simulink library "Feuchtesimulation_Lib"  (R2018b)
settings: Solver=VariableStepAuto  StartTime=0.0  StopTime=10.0  RelTol=1e-3
undefined symbols (not defined in the file or in its folder): A_Kat0, A_Mantel_Kat0, Ads_AusnutzungsFaktor, adsorptionsenthalpie, AIR_mw, beladungskennfeld, c_edelstahl, c_Isomatte, deltaH_verd, DiscIntNeverNeededParam, H2O_mw, Kat0_Anzahl_Zonen, Kond_AusnutzungsFaktor, Kond_KL_Faktor_, KondVerd_KLKF_mf_StSt_kgps, l_Kat0, m_Canning_Kat0, m_h2o_kat0_ads, m_h2o_kat0_kond, m_Isolierung_Kat0, m_zeolith_kat0_zone, m_zKat0, Mat_Kat0, mGas_imRohrabschnitt_kg, mZeo_UnterDerZeo0angenommenWird, p_dsat, R_sLuft, rate_k_verd, Rohr1, RTh_Brick_Iso_Kat0, RTh_Iso_Canning_Kat0, Sensor0, SensorIn, switch_TInit_Tstart_bei_true_sonst_TInitAusMessung, T_start, Tk0_1, ts, Verd_KF_Dampfdruck_StSt, Verd_KL_Faktor, waermekapazitaet_luft, waermekapazitaet_wasser_fluessig, waermekapazitaet_wasser_gasfoermig, WuezRohr_Dynamikfaktor
libraries: simulink x5, $bdroot x3
(part 2 of 2)

== system Feuchtesimulation_Lib/Brick/Adsorption Kondensation/Eingangskorrektur Adsorption ==
  note: Da das Adsorptionsmodell nachgeschalten ist kann es sein, dass das Model Wasser
      | "austragen" möchte obwohl kein Kondenzwasser verfügbar ist.
      |
      | Wenn m_Kond<=0 und deltaS<0 (sF kleiner als maximale Feuchte), dann ist der
      | Ausgang 0
  Delta S Kondensation : Inport
  Masse Kondensation : Inport  Port=2
  Constant2 : Constant  Value=0
  MATLAB Function : MATLAB Function  TreatAsAtomicUnit=on
  Switch : Switch  Criteria=u2 > Threshold
  Korrektur Adsorption Eingang : Outport
  wires:
  Delta S Kondensation/1 -> Switch/3, MATLAB Function/1(u1)
  Constant2/1 -> Switch/1
  MATLAB Function/1(y) -> Switch/2
  Masse Kondensation/1 -> MATLAB Function/2(u2)
  Switch/1 -> Korrektur Adsorption Eingang/1

== system Feuchtesimulation_Lib/Brick/Adsorption Kondensation/Kondensation ==
  note: Berechnet die Maximale Feuchte über die Formel:
      | s_max = H2O_mw/AIR_mw*p_dsat/(p-(1-H2O_mw/AIR_mw)*p_dsat)
      |
      | Der sättigungsdampfdruck wird über das Kennfeld bestimmt
  Bauteiltemperatur [°C] : Inport
  Druck [mbar] : Inport  Port=2
  spezifische Feuchte [kg/kg] : Inport  Port=3
  1-D Lookup Table : Lookup_n-D  NumberOfTableDimensions=1  BreakpointsForDimension1=p_dsat.T  Table=p_dsat.p  ExtrapMethod=Clip  InternalRulePriority=Speed  RndMeth=Simplest  InputSameDT=on
  Gain : Gain  Gain=Kond_AusnutzungsFaktor
  Limit Sättigungsdampfdruck : Subsystem
  Maximale spez Luftf. : MATLAB Function  TreatAsAtomicUnit=on
  Sat 0-1 : Saturate  UpperLimit=1  LowerLimit=0
  Sum : Sum  Inputs=|+-
  Ueberschuss spez. Feuchte [kg/kg] : Outport
  wires:
  1-D Lookup Table/1 -> Limit Sättigungsdampfdruck/2(Sättigungsdampfdruck [mbar])
  Bauteiltemperatur [°C]/1 -> 1-D Lookup Table/1
  Maximale spez Luftf./1(s_max) -> Sat 0-1/1
  Sum/1 -> Gain/1
  spezifische Feuchte [kg/kg]/1 -> Sum/1
  Sat 0-1/1 -> Sum/2
  Limit Sättigungsdampfdruck/1(Sättigungsdampfdruck Limitiert [mbar]) -> Maximale spez Luftf./2(p_dsat_mbar)
  Druck [mbar]/1 -> Limit Sättigungsdampfdruck/1(Druck [mbar]), Maximale spez Luftf./1(p_mbar)
  Gain/1 -> Ueberschuss spez. Feuchte [kg/kg]/1

== system Feuchtesimulation_Lib/Brick/Adsorption Kondensation/Theta Max  ==
  note: Ermittelt die aktuell maximal mögliche Wasserbeladung des Zeolithmasse
      | in Abhängigkeit der Temperatur und des Wasserdampfpartialdrucks
  Bauteiltemperatur [°C] : Inport
  Druck in [mbar] : Inport  Port=2
  spezifische Feuchte [kg/kg] : Inport  Port=3
  % to 1 : Gain  Gain=0.01
  2-D Lookup Table : Lookup_n-D  BreakpointsForDimension1=beladungskennfeld.Temp_C  BreakpointsForDimension2=beladungskennfeld.pSat_Pa  Table=beladungskennfeld.Beladung_prz  ExtrapMethod=Clip  InternalRulePriority=Speed  RndMeth=Simplest  InputSameDT=on
  S to E : Subsystem  AncestorBlock=Kats/S to E
  mbar to pa : Gain  Gain=100
  Theta_max [kg/kg] : Outport
  wires:
  mbar to pa/1 -> 2-D Lookup Table/2
  % to 1/1 -> Theta_max [kg/kg]/1
  2-D Lookup Table/1 -> % to 1/1
  spezifische Feuchte [kg/kg]/1 -> S to E/2(s)
  Druck in [mbar]/1 -> S to E/1(p_mbar)
  Bauteiltemperatur [°C]/1 -> 2-D Lookup Table/1
  S to E/1(e_mbar) -> mbar to pa/1

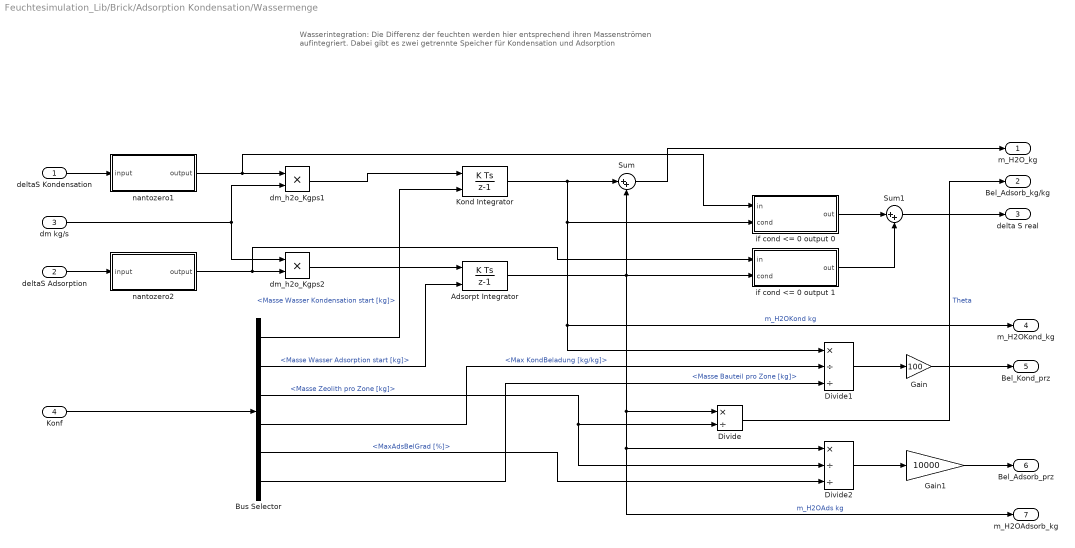
== system Feuchtesimulation_Lib/Brick/Adsorption Kondensation/Wassermenge  ==
  note: Wasserintegration:
      | Die Differenz der feuchten werden hier entsprechend ihren Massenströmen aufintegriert.
      | Dabei gibt es zwei getrennte Speicher für Kondensation und Adsorption
  deltaS Kondensation : Inport
  deltaS Adsorption : Inport  Port=2
  dm kg/s : Inport  Port=3
  Konf : Inport  Port=4
  Adsorpt Integrator : DiscreteIntegrator  InitialConditionSource=external  SampleTime=ts  LimitOutput=on  LowerSaturationLimit=0  ICPrevOutput=DiscIntNeverNeededParam  ICPrevScaledInput=DiscIntNeverNeededParam
  Bus Selector : BusSelector  OutputSignals=Masse Wasser Kondensation start [kg],Masse Wasser Adsorption start [kg],Masse Zeolith pro Zone [kg],Material Bauteil.Max KondBeladung [kg/kg],Material Bauteil.MaxAdsBelGrad [%],Masse Bauteil pro Zone [kg]
  Divide : Product  Inputs=*/
  Divide1 : Product  Inputs=*//
  Divide2 : Product  Inputs=*//
  Gain : Gain  Gain=100
  Gain1 : Gain  Gain=10000
  Kond Integrator : DiscreteIntegrator  InitialConditionSource=external  SampleTime=ts  LimitOutput=on  LowerSaturationLimit=0  ICPrevOutput=DiscIntNeverNeededParam  ICPrevScaledInput=DiscIntNeverNeededParam
  Sum : Sum  Inputs=|++
  Sum1 : Sum  Inputs=|++
  dm_h2o_Kgps1 : Product
  dm_h2o_Kgps2 : Product
  if cond <= 0 output 0 : Subsystem
  if cond <= 0 output 1 : Subsystem
  nantozero1 : Subsystem
  nantozero2 : Subsystem
  m_H2O_kg : Outport
  Bel_Adsorb_kg/kg : Outport  Port=2
  delta S real : Outport  Port=3
  m_H2OKond_kg : Outport  Port=4
  Bel_Kond_prz : Outport  Port=5
  Bel_Adsorb_prz : Outport  Port=6
  m_H2OAdsorb_kg : Outport  Port=7
  wires:
  deltaS Kondensation/1 -> nantozero1/1(input)
  deltaS Adsorption/1 -> nantozero2/1(input)
  Bus Selector/3 -> Divide2/2, Divide/2  "<Masse Zeolith pro Zone [kg]>"
  Divide/1 -> Bel_Adsorb_kg/kg/1  "Theta"
  Sum/1 -> m_H2O_kg/1
  dm_h2o_Kgps1/1 -> Kond Integrator/1
  dm_h2o_Kgps2/1 -> Adsorpt Integrator/1
  dm kg/s/1 -> dm_h2o_Kgps1/2, dm_h2o_Kgps2/1
  Kond Integrator/1 -> Divide1/1, m_H2OKond_kg/1, if cond <= 0 output 0/2(cond), Sum/1  "m_H2OKond kg"
  Sum1/1 -> delta S real/1
  Adsorpt Integrator/1 -> if cond <= 0 output 1/2(cond), m_H2OAdsorb_kg/1, Divide2/1, Divide/1, Sum/2  "m_H2OAds kg"
  nantozero2/1(output) -> if cond <= 0 output 1/1(in), dm_h2o_Kgps2/2
  Konf/1 -> Bus Selector/1
  Bus Selector/2 -> Adsorpt Integrator/2  "<Masse Wasser Adsorption start [kg]>"
  Bus Selector/1 -> Kond Integrator/2  "<Masse Wasser Kondensation start [kg]>"
  if cond <= 0 output 0/1(out) -> Sum1/1
  if cond <= 0 output 1/1(out) -> Sum1/2
  Divide1/1 -> Gain/1
  Bus Selector/4 -> Divide1/2  "<Max KondBeladung [kg/kg]>"
  nantozero1/1(output) -> if cond <= 0 output 0/1(in), dm_h2o_Kgps1/1
  Bus Selector/5 -> Divide2/3  "<MaxAdsBelGrad [%]>"
  Gain/1 -> Bel_Kond_prz/1
  Divide2/1 -> Gain1/1
  Gain1/1 -> Bel_Adsorb_prz/1
  Bus Selector/6 -> Divide1/3  "<Masse Bauteil pro Zone [kg]>"

== system Feuchtesimulation_Lib/Brick/Enthalpiestrom ausgehend /kombinierte Wärmekapazität ==
  Spezifische Feuchte : Inport
  Constant : Constant
  Constant1 : Constant  Value=waermekapazitaet_wasser_gasfoermig
  Multiply : Product
  Multiply1 : Product
  Sum : Sum  Inputs=|+-
  Sum1 : Sum  Inputs=|++
  cp1 : Constant  Value=waermekapazitaet_luft
  kombinierte Wärmekapazität : Outport
  wires:
  Multiply/1 -> Sum1/2
  Sum/1 -> Multiply/1
  Constant/1 -> Sum/1
  Spezifische Feuchte/1 -> Sum/2, Multiply1/1
  Constant1/1 -> Multiply1/2
  cp1/1 -> Multiply/2
  Multiply1/1 -> Sum1/1
  Sum1/1 -> kombinierte Wärmekapazität/1

== system Feuchtesimulation_Lib/Brick/Enthalpiestrom eingehend /kombinierte Wärmekapazität ==
  Spezifische Feuchte : Inport
  Constant : Constant
  Constant1 : Constant  Value=waermekapazitaet_wasser_gasfoermig
  Multiply : Product
  Multiply1 : Product
  Sum : Sum  Inputs=|+-
  Sum1 : Sum  Inputs=|++
  cp1 : Constant  Value=waermekapazitaet_luft
  kombinierte Wärmekapazität : Outport
  wires:
  Multiply/1 -> Sum1/2
  Sum/1 -> Multiply/1
  Constant/1 -> Sum/1
  Spezifische Feuchte/1 -> Sum/2, Multiply1/1
  Constant1/1 -> Multiply1/2
  cp1/1 -> Multiply/2
  Multiply1/1 -> Sum1/1
  Sum1/1 -> kombinierte Wärmekapazität/1

== system Feuchtesimulation_Lib/Rohrwandabschnitt/Kondensation/Taupunkt ==
  note: Berechnet die Taupunkttemperatur abhängig von abs. Druck und Feuchte
      |
      | TP-Formel basiert auf Magnusformel für Sättigungsdampfdruck
      | (Gültigkeitsbereich -45 (unterkühltes Wasser) bis +60°C, passt aber gut für
      | alle sinnvoll überprüften Werte) und benötigt neben dem absoluten Druck
      | als Feuchtemaß das Mischungsverhältnis (mWasser/mtrockeneLuft, 0 - inf),
      | welches sF/(1-sF) ist.
  spezifische Feuchte [kg/kg] : Inport
  Druck [mbar] : Inport  Port=2
  0<x<=0.999 : Saturate  UpperLimit=0.999  LowerLimit=0
  1e-6<x<1e6 : Saturate  UpperLimit=1e6  LowerLimit=1e-6
  Constant2 : Constant
  MATLAB Function : MATLAB Function  TreatAsAtomicUnit=on
  Sum : Sum  Inputs=-+
  sF/(1-sF) : Product  Inputs=*/
  Taupunkt [°C] : Outport
  wires:
  MATLAB Function/1(T_tp) -> Taupunkt [°C]/1
  Druck [mbar]/1 -> MATLAB Function/2(p)
  Constant2/1 -> Sum/2
  Sum/1 -> sF/(1-sF)/2
  sF/(1-sF)/1 -> 1e-6<x<1e6/1  "Mischungsverhaeltnis x"
  0<x<=0.999/1 -> Sum/1, sF/(1-sF)/1
  spezifische Feuchte [kg/kg]/1 -> 0<x<=0.999/1
  1e-6<x<1e6/1 -> MATLAB Function/1(x)

== system Feuchtesimulation_Lib/Rohrwandabschnitt/Q Gas an Wand/dm_2_v ==
  dm_kg/s : Inport
  p_mbar : Inport  Port=2
  Tg_C : Inport  Port=3
  D_eff_m : Inport  Port=4
  A_Rohr_m2 : Product  Inputs=***
  Constant1 : Constant  Value=3.14/4
  Constant2 : Constant  Value=R_sLuft
  Pa : Gain  Gain=100
  degC --> K : Subsystem
  m/A/rho : Product  Inputs=*//
  rho : Product  Inputs=*//
  v_m/s : Outport
  wires:
  dm_kg/s/1 -> m/A/rho/1
  rho/1 -> m/A/rho/2  "kg/m3"
  A_Rohr_m2/1 -> m/A/rho/3
  m/A/rho/1 -> v_m/s/1
  Constant2/1 -> rho/3
  degC --> K/1(K) -> rho/2
  p_mbar/1 -> Pa/1
  Pa/1 -> rho/1
  D_eff_m/1 -> A_Rohr_m2/2, A_Rohr_m2/1
  Constant1/1 -> A_Rohr_m2/3
  Tg_C/1 -> degC --> K/1(degC)

== system Feuchtesimulation_Lib/Brick/Adsorption Kondensation/Kondensation/Limit Sättigungsdampfdruck ==
  note: Hier wird der Maximale Sättigungsdampfdruck limitiert, da sonst in der
      | berechnung eine Singularität auftritt. Ist der Sättigungsdampfdruck gleich
      | dem Druck, ist der maximale Feuchtegehalt erreicht.
  Druck [mbar] : Inport
  Sättigungsdampfdruck [mbar] : Inport  Port=2
  Sum : Sum  Inputs=|+-
  Switch : Switch  Criteria=u2 > Threshold  RndMeth=Simplest  SaturateOnIntegerOverflow=on  InputSameDT=on
  Sättigungsdampfdruck Limitiert [mbar] : Outport
  wires:
  Druck [mbar]/1 -> Switch/3, Sum/1
  Sättigungsdampfdruck [mbar]/1 -> Switch/1, Sum/2
  Sum/1 -> Switch/2
  Switch/1 -> Sättigungsdampfdruck Limitiert [mbar]/1

== system Feuchtesimulation_Lib/Brick/Adsorption Kondensation/Theta Max /S to E ==
  p_mbar : Inport
  s : Inport  Port=2
  Constant : Constant  Value=H2O_mw/AIR_mw
  Divide : Product  Inputs=*/
  Multiply : Product
  Multiply1 : Product
  Sum : Sum  Inputs=++-
  e_mbar : Outport
  wires:
  Divide/1 -> e_mbar/1
  Sum/1 -> Divide/2
  Constant/1 -> Multiply1/2, Sum/2
  Multiply1/1 -> Sum/3
  Multiply/1 -> Divide/1
  p_mbar/1 -> Multiply/1
  s/1 -> Multiply/2, Sum/1, Multiply1/1

== system Feuchtesimulation_Lib/Brick/Adsorption Kondensation/Wassermenge /if cond <= 0 output 0 ==
  in : Inport
  cond : Inport  Port=2
  Constant : Constant  Value=0
  Switch : Switch  Criteria=u2 > Threshold  RndMeth=Simplest  SaturateOnIntegerOverflow=on  InputSameDT=on
  out : Outport
  wires:
  cond/1 -> Switch/2
  Switch/1 -> out/1
  in/1 -> Switch/1
  Constant/1 -> Switch/3

== system Feuchtesimulation_Lib/Brick/Adsorption Kondensation/Wassermenge /if cond <= 0 output 1 ==
  in : Inport
  cond : Inport  Port=2
  Constant : Constant  Value=0
  Switch : Switch  Criteria=u2 > Threshold  RndMeth=Simplest  SaturateOnIntegerOverflow=on  InputSameDT=on
  out : Outport
  wires:
  cond/1 -> Switch/2
  Switch/1 -> out/1
  in/1 -> Switch/1
  Constant/1 -> Switch/3

== system Feuchtesimulation_Lib/Brick/Adsorption Kondensation/Wassermenge /nantozero1 ==
  input : Inport
  IsNaN : RelationalOperator  Operator=isNaN  OutDataTypeStr=boolean  RndMeth=Simplest
  Switch : Switch  Criteria=u2 > Threshold
  Zero : Constant  Value=0  OutDataTypeStr=Inherit: Inherit via back propagation
  output : Outport
  wires:
  Switch/1 -> output/1
  IsNaN/1 -> Switch/2
  input/1 -> IsNaN/1, Switch/3
  Zero/1 -> Switch/1

== system Feuchtesimulation_Lib/Brick/Adsorption Kondensation/Wassermenge /nantozero2 ==
  input : Inport
  IsNaN : RelationalOperator  Operator=isNaN  OutDataTypeStr=boolean  RndMeth=Simplest
  Switch : Switch  Criteria=u2 > Threshold
  Zero : Constant  Value=0  OutDataTypeStr=Inherit: Inherit via back propagation
  output : Outport
  wires:
  Switch/1 -> output/1
  IsNaN/1 -> Switch/2
  input/1 -> IsNaN/1, Switch/3
  Zero/1 -> Switch/1

== system Feuchtesimulation_Lib/Rohrwandabschnitt/Q Gas an Wand/dm_2_v/degC --> K ==
  degC : Inport
  Constant3 : Constant  Value=273
  Sum : Sum
  K : Outport
  wires:
  Constant3/1 -> Sum/2
  Sum/1 -> K/1
  degC/1 -> Sum/1

== matlab function Feuchtesimulation_Lib/sFmax@Temp1 ==
  data: p_mbar input; sFmax output; Temp_degC input
function sFmax = sF_Saettigung(p_mbar,Temp_degC)
%#codegen
k1 = 6.112;     % hPa nach Magnusformel
k2 = 17.62;
k3 = 243.12;
p_Saettigung_mbar = k1 * exp(k2*Temp_degC / (k3+Temp_degC));
if (p_Saettigung_mbar>p_mbar) 
    p_Saettigung_mbar=p_mbar;
end
sFmax = 0.622*p_Saettigung_mbar / (p_mbar - 0.378*p_Saettigung_mbar);          % diese Formel ist im Gegensatz zur Magnusformel in SI, hier wird weils geht trotzdem mit mbar weitergerechnet
sFmax = min(max(sFmax,0),1);

== matlab function Feuchtesimulation_Lib/Rohrwandabschnitt/Kondensation/sFmax@Temp1 ==
  data: p_mbar input; sFmax output; Temp_degC input
function sFmax = sF_Saettigung(p_mbar,Temp_degC)
%#codegen
k1 = 6.112;     % hPa nach Magnusformel
k2 = 17.62;
k3 = 243.12;
p_Saettigung_mbar = k1 * exp(k2*Temp_degC / (k3+Temp_degC));
if (p_Saettigung_mbar>p_mbar) 
    p_Saettigung_mbar=p_mbar;
end
sFmax = 0.622*p_Saettigung_mbar / (p_mbar - 0.378*p_Saettigung_mbar);          % diese Formel ist im Gegensatz zur Magnusformel in SI, hier wird weils geht trotzdem mit mbar weitergerechnet
sFmax = min(max(sFmax,0),1);

== matlab function Feuchtesimulation_Lib/Rohrwandabschnitt/Kondensation/sFmax@Temp2 ==
  data: p_mbar input; sFmax output; Temp_degC input
function sFmax = sF_Saettigung(p_mbar,Temp_degC)
%#codegen
k1 = 6.112;     % hPa nach Magnusformel
k2 = 17.62;
k3 = 243.12;
p_Saettigung_mbar = k1 * exp(k2*Temp_degC / (k3+Temp_degC));
if (p_Saettigung_mbar>p_mbar) 
    p_Saettigung_mbar=p_mbar;
end
sFmax = 0.622*p_Saettigung_mbar / (p_mbar - 0.378*p_Saettigung_mbar);          % diese Formel ist im Gegensatz zur Magnusformel in SI, hier wird weils geht trotzdem mit mbar weitergerechnet
sFmax = min(max(sFmax,0),1);

== matlab function Feuchtesimulation_Lib/Rohrwandabschnitt/Kondensation/pSaett ==
  data: p_mbar input; ps_mbar output; Temp_degC input
function ps_mbar = pS(p_mbar, Temp_degC)
%#codegen
k1 = 6.112;     % hPa nach Magnusformel
k2 = 17.62;
k3 = 243.12;
ps_mbar = k1 * exp(k2*Temp_degC / (k3+Temp_degC));
if (ps_mbar>p_mbar) 
    ps_mbar=p_mbar;
end

== matlab function Feuchtesimulation_Lib/MATLAB Function ==
  data: s input; x output
function x = stox(s)
%#codegen

x = s/(1-s);

== matlab function Feuchtesimulation_Lib/Brick/Adsorption Kondensation/Kondensation/Maximale spez Luftf. ==
  data: p_mbar input; p_dsat_mbar input; s_max output
function s_max = fcn(p_mbar,p_dsat_mbar)
    H2O_mw = 18.02;
    AIR_mw = 28.96;     
s_max = H2O_mw/AIR_mw*p_dsat_mbar/(p_mbar-(1-H2O_mw/AIR_mw)*p_dsat_mbar);
% Grundsätzlich ist die Formel mit Pa konzipiert, funktioniert aber wegen
% der Form auch mit mbar und jeder anderen multiplikativen Einheit

== matlab function Feuchtesimulation_Lib/Brick/Adsorption Kondensation/Eingangskorrektur Adsorption/MATLAB Function ==
  data: u1 input; y output; u2 input
function y = condition(u1,u2)
    if(u1<0 && u2<=0)
        y = 1;
    else
        y = 0;
    end

== matlab function Feuchtesimulation_Lib/Alpha Gas Wand/MATLAB Function ==
  data: tf input; alpha output; v input; dgl input
function alpha = LuftTurbulent(tf,v,dgl)
%#codegen

alpha = (4.13 + 0.23*tf/100 - 0.0077*(tf/100)^2)*v^0.75/dgl^0.25;

== matlab function Feuchtesimulation_Lib/Rohrwandabschnitt/Kondensation/Taupunkt/MATLAB Function ==
  data: x input; T_tp output; p input
function T_tp = Taupunkt(x,p)
%#codegen
k1 = 6.112;     % hPa
k2 = 17.62;
k3 = 243.12;
T_tp = k3*log(x*p/((0.622+x)*k1))/(k2-log(x*p/((0.622+x)*k1)));     % "log" ist "ln"

== matlab function Feuchtesimulation_Lib/Sp. Luftfeuchtigkeit ==
  data: x input; s output
function s = xtos(x)

a=x*2;

s = (x/abs(x))*abs(x)/(abs(x)+1);
